simulink model "simulacion_tanqueAgua"  (R2026a)
settings: Solver=VariableStepAuto  StopTime=50
undefined symbols (not defined in the file): A, h0, Hmax, K, tStep

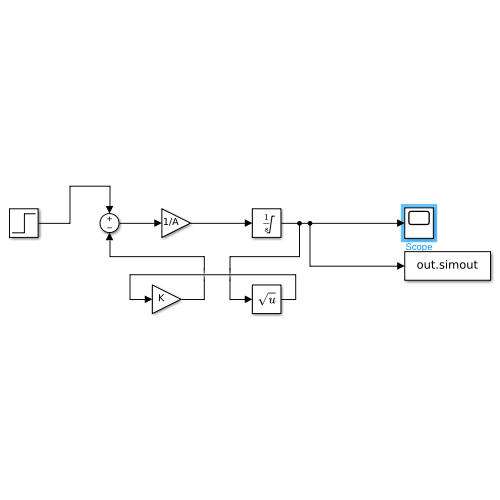
[thumbnail: Simulink's stored preview of the top-level diagram]
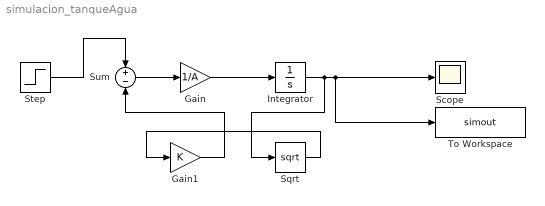
== system simulacion_tanqueAgua ==
  Gain : Gain  Gain=1/A
  Gain1 : Gain  Gain=K
  Integrator : Integrator  InitialCondition=h0  LimitOutput=on  UpperSaturationLimit=Hmax  LowerSaturationLimit=0
  Scope : Scope
      settings: ActiveDisplayYMinimum=4.7281085149454052  ActiveDisplayYMaximum=7.4470233654913542
  Sqrt : Sqrt
  Step : Step  Time=tStep  InitialValue=Qi0  FinalValue=Qi1  SampleTime=0
  Sum : Sum  Inputs=+-
  To Workspace : ToWorkspace  VariableName=simout  SaveFormat=Timeseries  SampleTime=-1
  wires:
  Step/1 -> Sum/1
  Sum/1 -> Gain/1
  Gain/1 -> Integrator/1
  Integrator/1 -> Sqrt/1, To Workspace/1, Scope/1
  Sqrt/1 -> Gain1/1
  Gain1/1 -> Sum/2
